simulink model "PI_illustration"  (R2024a)
settings: Solver=VariableStepAuto  StartTime=0.0  StopTime=20  RelTol=1e-3
libraries: slpidlib x1
settings Model: Creator=Lidia  LastModifiedBy=Lidia

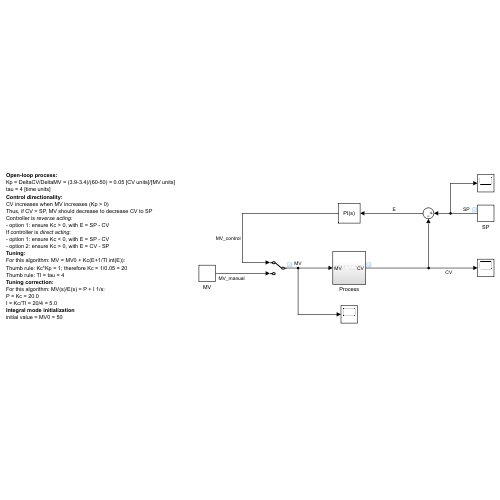
[thumbnail: Simulink's stored preview of the top-level diagram]
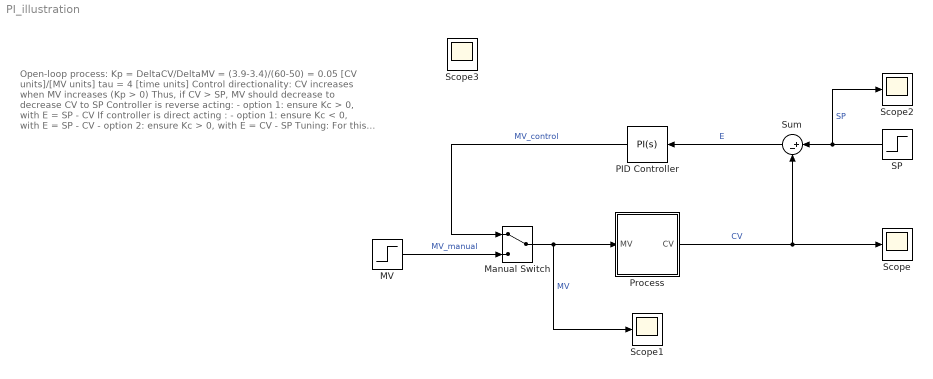
== system PI_illustration ==
  note: Open-loop process:
      | Kp = DeltaCV/DeltaMV = (3.9-3.4)/(60-50) = 0.05 [CV units]/[MV units]
      | tau = 4 [time units]
      | Control directionality:
      | CV increases when MV increases (Kp > 0)
      | Thus, if CV > SP, MV should decrease to decrease CV to SP
      | Controller is reverse acting:
      | - option 1: ensure Kc > 0, with E = SP - CV
      | If controller is direct acting :
      | - option 1: ensure Kc < 0, with E = SP - CV
      | - option 2: ensure Kc > 0, with E = CV - SP
      | Tuning:
      | For this algorithm: MV = MV0 + Kc(E+1/TI int(E)):
      | Thumb rule: Kc*Kp = 1; therefore Kc = 1/0.05 = 20
      | Thumb rule: TI = tau = 4
      | Tuning correction:
      | For this algorithm: MV(s)/E(s) = P + I 1/s:
      | P = Kc = 20.0
      | I = Kc/TI = 20/4 = 5.0
      | Integral mode initialization
      | initial value = MV0 = 50
  MV : Step  Before=50  After=60  SampleTime=0
  Manual Switch : ManualSwitch
  PID Controller : slpidlib/PID Controller  Controller=PI  Form=Parallel  TimeDomain=Continuous-time  UseExternalTs=off  SampleTime=-1  IntegratorMethod=Forward Euler  FilterMethod=Forward Euler  ControllerParametersSource=internal  P=20  I=4  UseKiTs=off  D=0  UseExternalDerivativeSource=off  N=100  UseFilter=on  TunerSelectOption=Transfer Function Based (PID Tuner App)  InitialConditionSource=internal  InitialConditionForIntegrator=50  InitialConditionForFilter=0  DifferentiatorICPrevScaledInput=0  ExternalReset=none  TrackingMode=off  Kt=1  LimitOutput=off  SatLimitsSource=external  UpperSaturationLimit=inf  LowerSaturationLimit=-inf  LinearizeAsGain=on  AntiWindupMode=none  Kb=1  LimitIntegrator=off  UpperIntegratorSaturationLimit=inf  LowerIntegratorSaturationLimit=-inf  POutMin=[]  POutMax=[]  IOutMin=[]  IOutMax=[]  DOutMin=[]  DOutMax=[]  NOutMin=[]  NOutMax=[]  SumOutMin=[]  SumOutMax=[]  SaturationOutMin=[]  SaturationOutMax=[]  PParamMin=[]  PParamMax=[]  IParamMin=[]  IParamMax=[]  DParamMin=[]  DParamMax=[]  NParamMin=[]  NParamMax=[]  KbParamMin=[]  KbParamMax=[]  KtParamMin=[]  KtParamMax=[]  KbOutMin=[]  KbOutMax=[]  KtOutMin=[]  KtOutMax=[]  IntegratorOutMin=[]  IntegratorOutMax=[]  FilterOutMin=[]  FilterOutMax=[]  SumI1OutMin=[]  SumI1OutMax=[]  SumI2OutMin=[]  SumI2OutMax=[]  SumI3OutMin=[]  SumI3OutMax=[]  SumI4OutMin=[]  SumI4OutMax=[]  SumDOutMin=[]  SumDOutMax=[]  DifferentiatorOutMin=[]  DifferentiatorOutMax=[]  FilterDiffOutCoefMin=[]  FilterDiffOutCoefMax=[]  ReciprocalOutMin=[]  ReciprocalOutMax=[]  SumDenOutMin=[]  SumDenOutMax=[]  SumNumOutMin=[]  SumNumOutMax=[]  DivideOutMin=[]  DivideOutMax=[]  UdiffTsProdOutMin=[]  UdiffTsProdOutMax=[]  NTsProdOutMin=[]  NTsProdOutMax=[]  UintegralTsProdOutMin=[]  UintegralTsProdOutMax=[]  UngainTsProdOutMin=[]  UngainTsProdOutMax=[]  ClampingZeroOutDataTypeStr=Inherit: Inherit via back propagation  ClampingZeroOutMin=[]  ClampingZeroOutMax=[]  FilterDenConstantOutDataTypeStr=Inherit: Inherit via back propagation  FilterDenConstantOutMin=[]  FilterDenConstantOutMax=[]  PCopyOutDataTypeStr=Inherit: Inherit via back propagation  PCopyOutMin=[]  PCopyOutMax=[]  NCopyOutDataTypeStr=Inherit: Inherit via back propagation  NCopyOutMin=[]  NCopyOutMax=[]  IntegratorContinuousStateAttributes=''  IntegratorStateMustResolveToSignalObject=off  IntegratorRTWStateStorageClass=Auto  FilterContinuousStateAttributes=''  FilterStateMustResolveToSignalObject=off  FilterRTWStateStorageClass=Auto  ParallelPVariant=InternalParameters  IdealPVariant=Disabled  IVariant=InternalParameters  DVariant=Disabled  IntegratorVariant=Continuous  SatVariant=Disabled  AWVariant=Passthrough  PCopyVariant=Disabled  TRVariant=Disabled  FdbkBlocksVariant=Forward  IdealPFdbkVariant=Disabled  SatFdbkVariant=Disabled  DerivativeFilterVariant=Disabled  NVariant=Disabled  NCopyVariant=Disabled_SignalSpec  FilterICVariant=Disabled  IntegratorICVariant=InternalICs  ExternalResetVariant=Disabled  TRSumVariant=Passthrough  SumFdbkVariant=Disabled  SumVariant=Sum_PI  TsampFilterVariant=InternalTs  TsampNgainVariant=Passthrough  TsampIntegralVariant=Disabled_SignalSpec  ExternalSaturationOutDataTypeStr=Inherit: Same as second input  DerivativeSourceVariant=Disabled
  Process : Subsystem
  SP : Step  Before=3.4  After=4.0  SampleTime=0
  Scope{,1..3} (4 alike) : Scope
  Sum : Sum  Inputs=|+-
  wires:
  Manual Switch/1 -> Scope1/1, Process/1(MV)  "MV"
  Process/1(CV) -> Scope/1, Sum/2  "CV"
  MV/1 -> Manual Switch/2  "MV_manual"
  SP/1 -> Scope2/1, Sum/1  "SP"
  Sum/1 -> PID Controller/1  "E"
  PID Controller/1 -> Manual Switch/1  "MV_control"

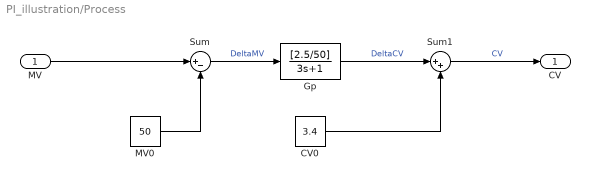
== system PI_illustration/Process ==
  MV : Inport
  CV0 : Constant  Value=3.4
  Gp : TransferFcn  Numerator=[2.5/50]  Denominator=[3 1]
  MV0 : Constant  Value=50
  Sum : Sum  Inputs=|+-
  Sum1 : Sum  Inputs=|++
  CV : Outport
  wires:
  Sum/1 -> Gp/1  "DeltaMV"
  CV0/1 -> Sum1/2
  Gp/1 -> Sum1/1  "DeltaCV"
  MV0/1 -> Sum/2
  MV/1 -> Sum/1
  Sum1/1 -> CV/1  "CV"
